simulink model "DC-motordrive"  (R2020a)
settings: Solver=VariableStepAuto  StartTime=0.0  StopTime=10.0  RelTol=1e-3
undefined symbols (not defined in the file or in its folder): b, kf, kic, kis, kpc, kps, r, Tmax, Tmin, Umax, Umin
settings Model: Creator=Dinesh Chandresh  LastModifiedBy=yk_yo

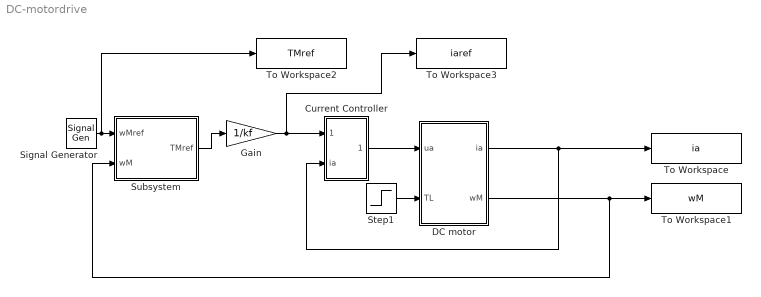
== system DC-motordrive ==
  Current Controller : Subsystem
  DC motor : Subsystem  mask{Ra=0.5, La=2.5e-3, kf=0.35, J=1e-3}
      mask prompts: Ra "Ra(ohm)"; La "La(H)"; kf "kf(Vs)"; J "J(Kgm^2)"
  Gain : Gain  Gain=1/kf
  Signal Generator : SignalGenerator  WaveForm=square  Frequency=100
  Step1 : Step  Time=0.3  After=7  SampleTime=0
  Subsystem : Subsystem
  To Workspace : ToWorkspace  VariableName=ia  SaveFormat=Timeseries  SampleTime=-1
  To Workspace1 : ToWorkspace  VariableName=wM  SaveFormat=Timeseries  SampleTime=-1
  To Workspace2 : ToWorkspace  VariableName=TMref  SaveFormat=Timeseries  SampleTime=-1
  To Workspace3 : ToWorkspace  VariableName=iaref  SaveFormat=Timeseries  SampleTime=-1
  wires:
  Step1/1 -> DC motor/2(TL)
  Current Controller/1(uaref) -> DC motor/1(ua)
  DC motor/1(ia) -> Current Controller/2(ia), To Workspace/1
  DC motor/2(wM) -> Subsystem/2(wM), To Workspace1/1
  Gain/1 -> To Workspace3/1, Current Controller/1(iaref)
  Signal Generator/1 -> To Workspace2/1, Subsystem/1(wMref)
  Subsystem/1(TMref) -> Gain/1

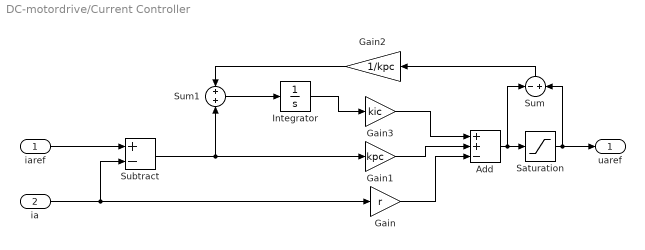
== system DC-motordrive/Current Controller ==
  iaref : Inport
  ia : Inport  Port=2
  Add : Sum  Inputs=++-
  Gain : Gain  Gain=r
  Gain1 : Gain  Gain=kpc
  Gain2 : Gain  Gain=1/kpc
  Gain3 : Gain  Gain=kic
  Integrator : Integrator
  Saturation : Saturate  UpperLimit=Umax  LowerLimit=Umin
  Subtract : Sum  Inputs=+-
  Sum : Sum  Inputs=-+
  Sum1 : Sum
  uaref : Outport
  wires:
  iaref/1 -> Subtract/1
  Add/1 -> Sum/1, Saturation/1
  Saturation/1 -> uaref/1, Sum/2
  Gain1/1 -> Add/2
  Subtract/1 -> Gain1/1, Sum1/2
  Gain/1 -> Add/3
  Gain2/1 -> Sum1/1
  ia/1 -> Gain/1, Subtract/2
  Sum/1 -> Gain2/1
  Gain3/1 -> Add/1
  Integrator/1 -> Gain3/1
  Sum1/1 -> Integrator/1

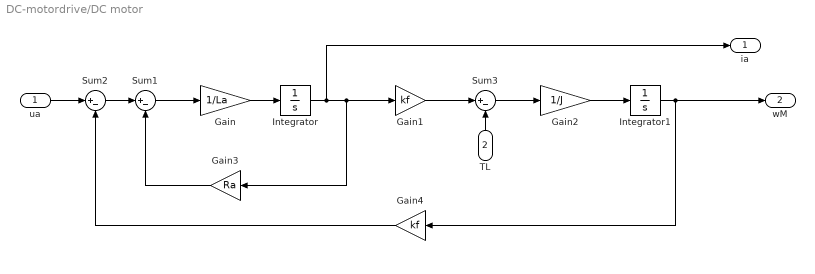
== system DC-motordrive/DC motor ==
  ua : Inport
  TL : Inport  Port=2
  Gain : Gain  Gain=1/La
  Gain1 : Gain  Gain=kf
  Gain2 : Gain  Gain=1/J
  Gain3 : Gain  Gain=Ra
  Gain4 : Gain  Gain=kf
  Integrator : Integrator
  Integrator1 : Integrator
  Sum1 : Sum  Inputs=|+-
  Sum2 : Sum  Inputs=|+-
  Sum3 : Sum  Inputs=|+-
  ia : Outport
  wM : Outport  Port=2
  wires:
  Integrator/1 -> ia/1, Gain3/1, Gain1/1
  Gain2/1 -> Integrator1/1
  TL/1 -> Sum3/2
  Gain/1 -> Integrator/1
  Integrator1/1 -> Gain4/1, wM/1
  Gain3/1 -> Sum1/2
  ua/1 -> Sum2/1
  Sum2/1 -> Sum1/1
  Sum1/1 -> Gain/1
  Sum3/1 -> Gain2/1
  Gain4/1 -> Sum2/2
  Gain1/1 -> Sum3/1

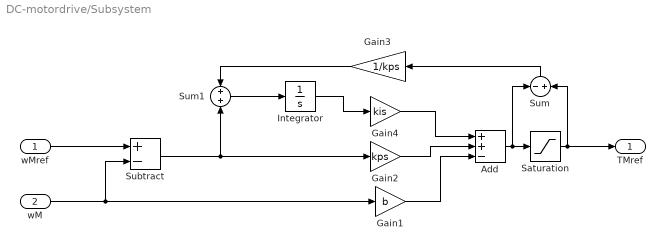
== system DC-motordrive/Subsystem ==
  wMref : Inport
  wM : Inport  Port=2
  Add : Sum  Inputs=++-
  Gain1 : Gain  Gain=b
  Gain2 : Gain  Gain=kps
  Gain3 : Gain  Gain=1/kps
  Gain4 : Gain  Gain=kis
  Integrator : Integrator
  Saturation : Saturate  UpperLimit=Tmax  LowerLimit=Tmin
  Subtract : Sum  Inputs=+-
  Sum : Sum  Inputs=-+
  Sum1 : Sum
  TMref : Outport
  wires:
  Saturation/1 -> TMref/1, Sum/2
  Sum1/1 -> Integrator/1
  Sum/1 -> Gain3/1
  wM/1 -> Gain1/1, Subtract/2
  Add/1 -> Sum/1, Saturation/1
  Subtract/1 -> Gain2/1, Sum1/2
  Gain1/1 -> Add/3
  wMref/1 -> Subtract/1
  Gain3/1 -> Sum1/1
  Gain4/1 -> Add/1
  Integrator/1 -> Gain4/1
  Gain2/1 -> Add/2
